simulink library "simeventsqueue2"  (Simulink 7.5)
settings: Solver=ode45  SolverMode=SingleTasking  StartTime=0.0  StopTime=10.0  RelTol=1e-3
undefined symbols (not defined in the file or in its folder): des_support, gcbh
settings Model: Creator=mclune  LastModifiedBy=ywu  ExtModeAutoUpdateStatusClock=off

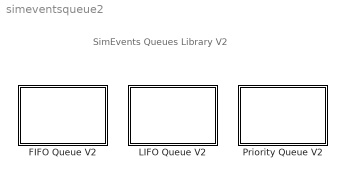
== system simeventsqueue2 ==
  note: SimEvents Queues Library V2
  FIFO Queue V2 : Subsystem  Priority=1  LoadFcn=des_support('desLoadFcn',gcbh)  StartFcn=des_support('desStartFcn',gcbh)  StopFcn=des_support('desStopFcn',gcbh)  mask(FIFO Queue V2){Capacity=25, EnableTOPort=off, StatNumberDeparted=Off, StatNumberInBlock=Off, StatPendingEntity=Off, StatAverageWait=Off, StatAverageQueueLength=Off, StatNumberTimedout=Off}
      mask prompts: EnableTOPort "Enable TO port for timed-out entities"; StatNumberDeparted "Number of entities departed, #d:"; StatNumberInBlock "Number of entities in queue, #n:"; StatPendingEntity "Status of pending entity departure, pe:"; StatAverageWait "Average wait, w:"; StatAverageQueueLength "Average queue length, len:"; StatNumberTimedout "Number of entities timed-out, #to:"
      mask help: Store entities in first-in-first-out sequence for an undetermined length of time. The Capacity parameter is the number of entities the queue can hold.
      mask init:
      | des_basicqueuemaskv2(gcb,'init','apply')
      settings: CopyFcn=des_support('desCopyFcn',gcbh)  DeleteFcn=des_support('desDeleteFcn',gcbh)  UndoDeleteFcn=des_support('desUndoDeleteFcn',gcbh)  ModelCloseFcn=des_support('desModelCloseFcn',gcbh)  PreSaveFcn=des_support('desPreSaveFcn',gcbh)  PostSaveFcn=des_support('desPostSaveFcn',gcbh)  NameChangeFcn=des_support('desNameChangeFcn',gcbh)  CloseFcn=des_support('desCloseFcn',gcbh)  ErrorFcn=des_error_redirect
      mask Help: helpview(simeventsbhelp)
      mask StyleString: edit,checkbox,popup(Off|On|Upon stop or pause),popup(Off|On|Upon stop or pause),popup(Off|On),popup(Off|On|Upon stop or pause),popup(Off|On|Upon stop or pause),popup(Off|On|Upon stop or pause)
      mask CallbackString: |des_basicqueuemaskv2(gcb,'cbEnableTOPort','noapply');|des_basicqueuemaskv2(gcb,'cbStatNumberDeparted','noapply');|des_basicqueuemaskv2(gcb,'cbStatNumberInBlock','noapply');||des_basicqueuemaskv2(gcb,'cbWait','noapply');|des_basicqueuemaskv2(gcb,'cbStatAverageQueueLength','noapply');|des_basicqueuemaskv2(gcb,'cbStatNumberTimedout','noapply');
      mask TabNameString: FIFO Queue,Timeout,Statistics,Statistics,Statistics,Statistics,Statistics,Statistics
      mask Display:
      | image(des_iconLoad('queueFIFO.jpg'),'center');
      | port_label('LConn',1,'IN');
      | port_label('RConn',1,'OUT');
  LIFO Queue V2 : Subsystem  Priority=1  LoadFcn=des_support('desLoadFcn',gcbh)  StartFcn=des_support('desStartFcn',gcbh)  StopFcn=des_support('desStopFcn',gcbh)  mask(LIFO Queue V2){Capacity=25, EnableTOPort=off, StatNumberDeparted=Off, StatNumberInBlock=Off, StatPendingEntity=Off, StatAverageWait=Off, StatAverageQueueLength=Off, StatNumberTimedout=Off}
      mask prompts: EnableTOPort "Enable TO port for timed-out entities"; StatNumberDeparted "Number of entities departed, #d:"; StatNumberInBlock "Number of entities in queue, #n:"; StatPendingEntity "Status of pending entity departure, pe:"; StatAverageWait "Average wait, w:"; StatAverageQueueLength "Average queue length, len:"; StatNumberTimedout "Number of entities timed-out, #to:"
      mask help: Store entities in last-in-first-out sequence for an undetermined length of time. The Capacity parameter is the number of entities the queue can hold.
      mask init:
      | des_lifoqueuemaskv2(gcb,'init','apply')
      settings: CopyFcn=des_support('desCopyFcn',gcbh)  DeleteFcn=des_support('desDeleteFcn',gcbh)  UndoDeleteFcn=des_support('desUndoDeleteFcn',gcbh)  ModelCloseFcn=des_support('desModelCloseFcn',gcbh)  PreSaveFcn=des_support('desPreSaveFcn',gcbh)  PostSaveFcn=des_support('desPostSaveFcn',gcbh)  NameChangeFcn=des_support('desNameChangeFcn',gcbh)  CloseFcn=des_support('desCloseFcn',gcbh)  ErrorFcn=des_error_redirect
      mask Help: helpview(simeventsbhelp)
      mask StyleString: edit,checkbox,popup(Off|On|Upon stop or pause),popup(Off|On|Upon stop or pause),popup(Off|On),popup(Off|On|Upon stop or pause),popup(Off|On|Upon stop or pause),popup(Off|On|Upon stop or pause)
      mask CallbackString: |des_lifoqueuemaskv2(gcb,'cbEnableTOPort','noapply');|des_lifoqueuemaskv2(gcb,'cbStatNumberDeparted','noapply');|des_lifoqueuemaskv2(gcb,'cbStatNumberInBlock','noapply');||des_lifoqueuemaskv2(gcb,'cbWait','noapply');|des_lifoqueuemaskv2(gcb,'cbStatAverageQueueLength','noapply');|des_lifoqueuemaskv2(gcb,'cbStatNumberTimedout','noapply');
      mask TabNameString: LIFO Queue,Timeout,Statistics,Statistics,Statistics,Statistics,Statistics,Statistics
      mask Display:
      | image(des_iconLoad('queueLIFO.jpg'),'center');
      | port_label('LConn',1,'IN');
      | port_label('RConn',1,'OUT');
  Priority Queue V2 : Subsystem  Priority=1  LoadFcn=des_support('desLoadFcn',gcbh)  StartFcn=des_support('desStartFcn',gcbh)  StopFcn=des_support('desStopFcn',gcbh)  mask(Priority Queue V2){Capacity=25, SortingAttributeName=PriorityAttributeName, SortingDirection=Ascending, EnableTOPort=off, StatNumberDeparted=Off, StatNumberInBlock=Off, StatPendingEntity=Off, StatAverageWait=Off, StatAverageQueueLength=Off, StatNumberTimedout=Off}
      mask prompts: SortingAttributeName "Sorting attribute name:"; SortingDirection "Sorting direction:"; EnableTOPort "Enable TO port for timed-out entities"; StatNumberDeparted "Number of entities departed, #d:"; StatNumberInBlock "Number of entities in queue, #n:"; StatPendingEntity "Status of pending entity departure, pe:"; StatAverageWait "Average wait time, w:"; StatAverageQueueLength "Average queue length, len:"; StatNumberTimedout "Number of entities timed-out:"
      mask help: Store entities in sorted sequence for an undetermined length of time. The Capacity parameter is the number of entities the queue can hold. The queue sorts entities according to the values of the specified attribute, in either ascending or descending order.
      mask init:
      | des_priorityqueuemaskv2(gcb,'init','apply')
      settings: CopyFcn=des_support('desCopyFcn',gcbh)  DeleteFcn=des_support('desDeleteFcn',gcbh)  UndoDeleteFcn=des_support('desUndoDeleteFcn',gcbh)  ModelCloseFcn=des_support('desModelCloseFcn',gcbh)  PreSaveFcn=des_support('desPreSaveFcn',gcbh)  PostSaveFcn=des_support('desPostSaveFcn',gcbh)  NameChangeFcn=des_support('desNameChangeFcn',gcbh)  CloseFcn=des_support('desCloseFcn',gcbh)  ErrorFcn=des_error_redirect
      mask Help: helpview(simeventsbhelp)
      mask StyleString: edit,edit,popup(Ascending|Descending),checkbox,popup(Off|On|Upon stop or pause),popup(Off|On|Upon stop or pause),popup(Off|On),popup(Off|On|Upon stop or pause),popup(Off|On|Upon stop or pause),popup(Off|On|Upon stop or pause)
      mask CallbackString: |||des_priorityqueuemaskv2(gcb,'cbEnableTOPort','noapply');|des_priorityqueuemaskv2(gcb,'cbStatNumberDeparted','noapply');|des_priorityqueuemaskv2(gcb,'cbStatNumberInBlock','noapply');||des_priorityqueuemaskv2(gcb,'cbWait','noapply');|des_priorityqueuemaskv2(gcb,'cbStatAverageQueueLength','noapply');|des_priorityqueuemaskv2(gcb,'cbStatNumberTimedout','noapply');
      mask TabNameString: Priority Queue,Priority Queue,Priority Queue,Timeout,Statistics,Statistics,Statistics,Statistics,Statistics,Statistics
      mask Display:
      | image(des_iconLoad('queuePriority.jpg'),'center');
      | port_label('LConn',1,'IN');
      | port_label('RConn',1,'OUT');

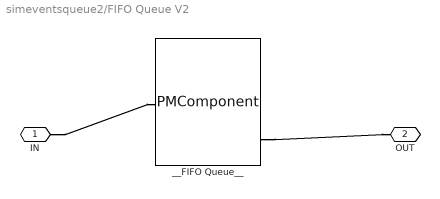
== system simeventsqueue2/FIFO Queue V2 ==
  __FIFO Queue__ : PMComponent  PhysicalDomain=simevents  SubClassName=DES_FIFOQUEUEV2  LeftPortType=desPortIn  RightPortType=desPortOut  LConnTagsString=DI  RConnTagsString=DO|DO|DO|DO|DO|DO|DO|DO
      mask Display:
      | port_label('LConn',1,'IN');
      | port_label('RConn',1,'#d');
      | port_label('RConn',2,'#n');
      | port_label('RConn',3,'pe');
      | port_label('RConn',4,'w');
      | port_label('RConn',5,'len');
      | port_label('RConn',6,'#to');
      | port_label('RConn',7,'OUT');
      | port_label('RConn',8,'TO');
  IN : PMIOPort  Port=1  Side=Left
  OUT : PMIOPort  Port=2  Side=Right
  connections:
  IN/RConn1 -- __FIFO Queue__/LConn1
  __FIFO Queue__/RConn7 -- OUT/RConn1

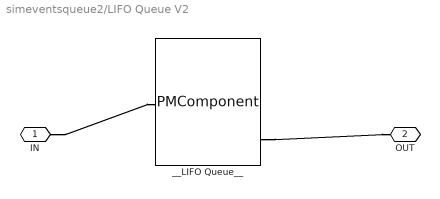
== system simeventsqueue2/LIFO Queue V2 ==
  __LIFO Queue__ : PMComponent  PhysicalDomain=simevents  SubClassName=DES_LIFOQUEUEV2  LeftPortType=desPortIn  RightPortType=desPortOut  LConnTagsString=DI  RConnTagsString=DO|DO|DO|DO|DO|DO|DO|DO
      mask Display:
      | port_label('LConn',1,'IN');
      | port_label('RConn',1,'#d');
      | port_label('RConn',2,'#n');
      | port_label('RConn',3,'pe');
      | port_label('RConn',4,'w');
      | port_label('RConn',5,'len');
      | port_label('RConn',6,'#to');
      | port_label('RConn',7,'OUT');
      | port_label('RConn',8,'TO');
  IN : PMIOPort  Port=1  Side=Left
  OUT : PMIOPort  Port=2  Side=Right
  connections:
  IN/RConn1 -- __LIFO Queue__/LConn1
  __LIFO Queue__/RConn7 -- OUT/RConn1

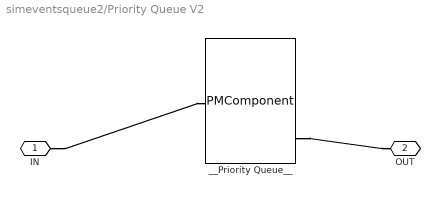
== system simeventsqueue2/Priority Queue V2 ==
  __Priority Queue__ : PMComponent  PhysicalDomain=simevents  SubClassName=DES_PRIORITYQUEUEV2  LeftPortType=desPortIn  RightPortType=desPortOut  LConnTagsString=DI  RConnTagsString=DO|DO|DO|DO|DO|DO|DO|DO
      mask Display:
      | port_label('LConn',1,'IN');
      | port_label('RConn',1,'#d');
      | port_label('RConn',2,'#n');
      | port_label('RConn',3,'pe');
      | port_label('RConn',4,'w');
      | port_label('RConn',5,'len');
      | port_label('RConn',6,'#to');
      | port_label('RConn',7,'OUT');
      | port_label('RConn',8,'TO');
  IN : PMIOPort  Port=1  Side=Left
  OUT : PMIOPort  Port=2  Side=Right
  connections:
  IN/RConn1 -- __Priority Queue__/LConn1
  __Priority Queue__/RConn7 -- OUT/RConn1
